simulink subsystem "ResonantLoad_SubSystem"  (R2020b)
settings: Solver=VariableStepAuto  StartTime=0.0  StopTime=10.0  RelTol=1e-3
undefined symbols (not defined in the file or in its folder): mld
settings Model: Creator=umberto  LastModifiedBy=umberto

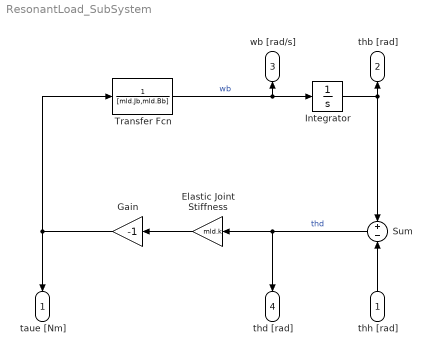
== system ResonantLoad_SubSystem ==
  thh [rad] : Inport
  Elastic Joint Stiffness : Gain  Gain=mld.k
  Gain : Gain  Gain=-1
  Integrator : Integrator
  Sum : Sum  Inputs=+|-
  Transfer Fcn : TransferFcn  Denominator=[mld.Jb,mld.Bb]
  taue [Nm] : Outport
  thb [rad] : Outport  Port=2
  wb [rad/s] : Outport  Port=3
  thd [rad] : Outport  Port=4
  wires:
  thh [rad]/1 -> Sum/2
  Sum/1 -> Elastic Joint Stiffness/1, thd [rad]/1  "thd"
  Elastic Joint Stiffness/1 -> Gain/1
  Gain/1 -> Transfer Fcn/1, taue [Nm]/1
  Transfer Fcn/1 -> Integrator/1, wb [rad/s]/1  "wb"
  Integrator/1 -> Sum/1, thb [rad]/1
